simulink model "PCIe_UserLogic_00"  (Simulink 7.6)
settings: Solver=ode45  StartTime=0.0  StopTime=10.0  RelTol=1e-3
PreLoadFcn:
  | SP605_TS  = 1/200e6;
  | SP605_CLK = SP605_TS*1e9;
  | USER_TS  = 1/200e6;
  | USER_CLK = USER_TS*1e9;
  | 
  | PCIE_TS   = 1/125e6;
  | PCIE_CLK = PCIE_TS*1e9;
  | 
  | P_Size = 32;
  | 
  | WR_LAT = 10 + round(P_Size*5/12);
InitFcn:
  | SP605_TS  = 1/200e6;
  | SP605_CLK = SP605_TS*1e9;
  | USER_TS  = 1/200e6;
  | USER_CLK = USER_TS*1e9;
  | 
  | PCIE_TS   = 1/125e6;
  | PCIE_CLK = PCIE_TS*1e9;
  | 
  | P_Size = 32;
  | 
  | WR_LAT = 10 + round(P_Size*5/12);
libraries: xbsIndex_r4 x341
(part 3 of 3)

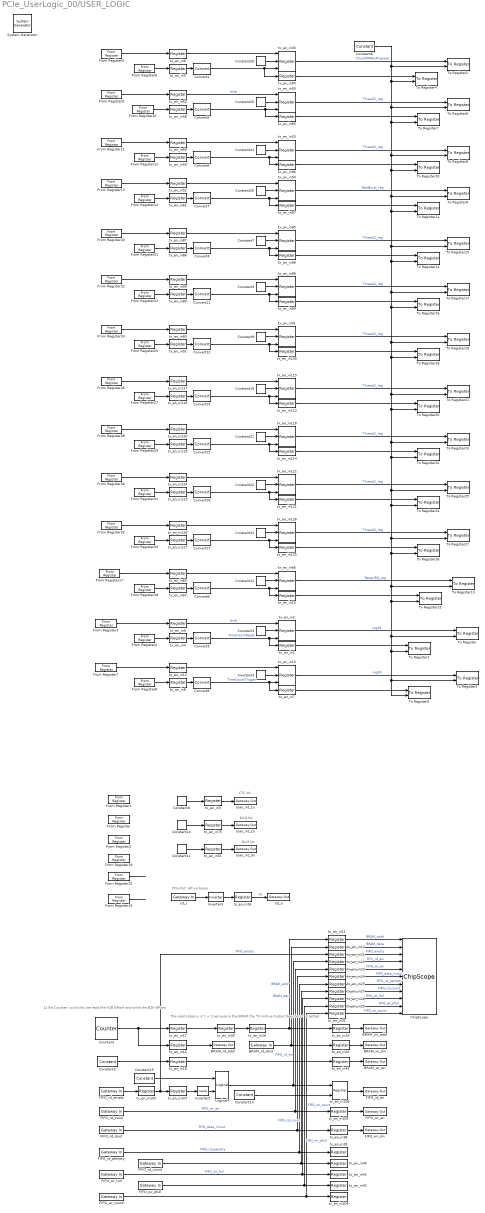
== system PCIe_UserLogic_00/USER_LOGIC ==
  note: The read Latency is 1 + 1 becouse
      | in the BRAM the "Primitive Output Registersr" is setted
  note: CTL bit
  note: DAQ bit
  note: DLM bit
  note: PCIe Rst: Attivo basso
  note: 12 Bit Counter:
      | cyclically we read the H2B BRam
      | and write the B2H BRam
  " System Generator" : xbsIndex_r4/ System Generator  Tag=genX  SystemSampleTime=-1  xilinxfamily=virtex6  part=xc6vlx240t  speed=-1  package=ff1156  synthesis_tool=XST  clock_wrapper=Clock Enables  directory=C:/Temp/Xilinx PCI Express/ML605_ISE13.3/MyUserLogic/UserLogic_00/top_level_1_PCIe_UserLogic_00_USER_LOGIC  proj_type=Project Navigator  Synth_file=XST Defaults  Impl_file=ISE Defaults  testbench=off  simulink_period=USER_TS  sysclk_period=USER_CLK  dcm_input_clock_period=5  incr_netlist=off  trim_vbits=Everywhere in SubSystem  dbl_ovrd=According to Block Masks  core_generation=According to Block Masks  run_coregen=off  deprecated_control=off  eval_field=0  block_type=sysgen
      settings: block_version=12.3
  BRAM_rd_addr : xbsIndex_r4/Gateway Out  hdl_port=on  timing_constraint=None  locs_specified=off  LOCs={}  block_type=gatewayout
      settings: infoedit="Gateway out block.  Converts Xilinx fixed point or floating-point type inputs into ouputs of type Simulink integer, double, or fixed point.<br><br>Hardware notes:  In hardware these blocks become top level output ports or are discarded, depending on how they are configured."  block_version=12.3
  BRAM_rd_dout : xbsIndex_r4/Gateway In  gui_display_data_type=Fixed-point  arith_type=Unsigned  n_bits=64  bin_pt=0  preci_type=Single  exp_width=8  frac_width=24  quantization="Round  (unbiased: +/- Inf)"  overflow=Saturate  period=USER_TS  dbl_ovrd=off  timing_constraint=None  locs_specified=off  LOCs={}  hdl_port=on  block_type=gatewayin
      settings: infoedit="Gateway in block.  Converts inputs of type Simulink integer, double and fixed point to  Xilinx fixed point type.<br><br>Hardware notes:  In hardware these blocks become top level input ports."  block_version=12.3
  BRAM_wr_addr : xbsIndex_r4/Gateway Out  hdl_port=on  timing_constraint=None  locs_specified=off  LOCs={}  block_type=gatewayout
      settings: infoedit="Gateway out block.  Converts Xilinx fixed point or floating-point type inputs into ouputs of type Simulink integer, double, or fixed point.<br><br>Hardware notes:  In hardware these blocks become top level output ports or are discarded, depending on how they are configured."  block_version=12.3
  BRAM_wr_din : xbsIndex_r4/Gateway Out  hdl_port=on  timing_constraint=None  locs_specified=off  LOCs={}  block_type=gatewayout
      settings: infoedit="Gateway out block.  Converts Xilinx fixed point or floating-point type inputs into ouputs of type Simulink integer, double, or fixed point.<br><br>Hardware notes:  In hardware these blocks become top level output ports or are discarded, depending on how they are configured."  block_version=12.3
  BRAM_wr_en : xbsIndex_r4/Gateway Out  hdl_port=on  timing_constraint=None  locs_specified=off  LOCs={}  block_type=gatewayout
      settings: infoedit="Gateway out block.  Converts Xilinx fixed point or floating-point type inputs into ouputs of type Simulink integer, double, or fixed point.<br><br>Hardware notes:  In hardware these blocks become top level output ports or are discarded, depending on how they are configured."  block_version=12.3
  ChipScope : xbsIndex_r4/ChipScope  num_trig_ports=11  current_port=0  show_trig_port=0  match_units=1  match_type=Basic  data_is_trigger=on  num_data_ports=1  data_depth=1024  SRL16s=on  add_bufg=on  match_type_t0=1  match_type_t1=1  match_type_t2=1  match_type_t3=1  match_type_t4=1  match_type_t5=1  match_type_t6=1  match_type_t7=1  match_type_t8=1  match_type_t9=1  match_type_t10=1  match_type_t11=1  match_type_t12=1  match_type_t13=1  match_type_t14=1  match_type_t15=1  match_units_t0=1  match_units_t1=1  match_units_t2=1  match_units_t3=1  match_units_t4=1  match_units_t5=1  match_units_t6=1  match_units_t7=1  match_units_t8=1  match_units_t9=1  match_units_t10=1  match_units_t11=1  match_units_t12=1  match_units_t13=1  match_units_t14=1  match_units_t15=1  dbl_ovrd=0  user_scan_chain=USER1  block_type=chipscope
      settings: infoedit="Enables run-time debugging and verification of signals by inserting ChipScope Pro ICON and ILA cores.<br><br>  Restrictions: <br>Only one ChipScope core can be instantiated in a System Generator design. A design or subsystem containing a ChipScope block must have at least one output port."
  Constant{1,3..4,7..12,19..26} (17 alike) : xbsIndex_r4/Constant  const=0  gui_display_data_type=Fixed-point  arith_type=Boolean  n_bits=32  bin_pt=0  preci_type=Single  exp_width=8  frac_width=24  explicit_period=on  period=USER_TS  equ=P=C  opselect=C  inp2=PCIN>>17  opr=+  inp1=P  carry=CIN  dbl_ovrd=off  block_type=constant
      settings: block_version=12.3
  Constant14 : xbsIndex_r4/Constant  const=1  gui_display_data_type=Fixed-point  arith_type=Boolean  n_bits=8  bin_pt=0  preci_type=Single  exp_width=8  frac_width=24  explicit_period=on  period=USER_TS  equ=P=C  opselect=C  inp2=PCIN>>17  opr=+  inp1=P  carry=CIN  dbl_ovrd=off  block_type=constant
      settings: block_version=12.3
  Constant15 : xbsIndex_r4/Constant  const=1  gui_display_data_type=Fixed-point  arith_type=Boolean  n_bits=8  bin_pt=0  preci_type=Single  exp_width=8  frac_width=24  explicit_period=on  period=USER_TS  equ=P=C  opselect=C  inp2=PCIN>>17  opr=+  inp1=P  carry=CIN  dbl_ovrd=off  block_type=constant
      settings: block_version=12.3
  Constant2 : xbsIndex_r4/Constant  const=255  gui_display_data_type=Fixed-point  arith_type=Unsigned  n_bits=8  bin_pt=0  preci_type=Single  exp_width=8  frac_width=24  explicit_period=on  period=USER_TS  equ=P=C  opselect=C  inp2=PCIN>>17  opr=+  inp1=P  carry=CIN  dbl_ovrd=off  block_type=constant
      settings: block_version=12.3
  Constant6 : xbsIndex_r4/Constant  const=1  gui_display_data_type=Fixed-point  arith_type=Boolean  n_bits=32  bin_pt=0  preci_type=Single  exp_width=8  frac_width=24  explicit_period=on  period=USER_TS  equ=P=C  opselect=C  inp2=PCIN>>17  opr=+  inp1=P  carry=CIN  dbl_ovrd=off  block_type=constant
      settings: block_version=12.3
  Convert{1,3..9,11..12,14..17} (14 alike) : xbsIndex_r4/Convert  gui_display_data_type=Fixed-point  arith_type=Boolean  n_bits=16  bin_pt=14  float_type=Single  exp_bits=8  fraction_bits=24  quantization=Truncate  overflow=Wrap  en=off  latency=0  dbl_ovrd=off  pipeline=off  block_type=convert
      settings: block_version=12.3
  Counter4 : xbsIndex_r4/Counter  cnt_type=Free Running  cnt_to=Inf  operation=Up  start_count=0  cnt_by_val=1  arith_type=Unsigned  n_bits=12  bin_pt=0  load_pin=off  rst=off  en=off  explicit_period=on  period=USER_TS  dbl_ovrd=off  use_behavioral_HDL=off  implementation=Fabric  block_type=counter
      settings: block_version=12.3
  FIFO_rd_count : xbsIndex_r4/Gateway In  gui_display_data_type=Fixed-point  arith_type=Unsigned  n_bits=15  bin_pt=0  preci_type=Single  exp_width=8  frac_width=24  quantization="Round  (unbiased: +/- Inf)"  overflow=Saturate  period=USER_TS  dbl_ovrd=off  timing_constraint=None  locs_specified=off  LOCs={}  hdl_port=on  block_type=gatewayin
      settings: infoedit="Gateway in block.  Converts inputs of type Simulink integer, double and fixed point to  Xilinx fixed point type.<br><br>Hardware notes:  In hardware these blocks become top level input ports."  block_version=12.3
  FIFO_rd_dout : xbsIndex_r4/Gateway In  gui_display_data_type=Fixed-point  arith_type=Unsigned  n_bits=72  bin_pt=0  preci_type=Single  exp_width=8  frac_width=24  quantization="Round  (unbiased: +/- Inf)"  overflow=Saturate  period=USER_TS  dbl_ovrd=off  timing_constraint=None  locs_specified=off  LOCs={}  hdl_port=on  block_type=gatewayin
      settings: infoedit="Gateway in block.  Converts inputs of type Simulink integer, double and fixed point to  Xilinx fixed point type.<br><br>Hardware notes:  In hardware these blocks become top level input ports."  block_version=12.3
  FIFO_rd_empty : xbsIndex_r4/Gateway In  gui_display_data_type=Fixed-point  arith_type=Boolean  n_bits=12  bin_pt=0  preci_type=Single  exp_width=8  frac_width=24  quantization="Round  (unbiased: +/- Inf)"  overflow=Saturate  period=USER_TS  dbl_ovrd=off  timing_constraint=None  locs_specified=off  LOCs={}  hdl_port=on  block_type=gatewayin
      settings: infoedit="Gateway in block.  Converts inputs of type Simulink integer, double and fixed point to  Xilinx fixed point type.<br><br>Hardware notes:  In hardware these blocks become top level input ports."  block_version=12.3
  FIFO_rd_en : xbsIndex_r4/Gateway Out  hdl_port=on  timing_constraint=None  locs_specified=off  LOCs={}  block_type=gatewayout
      settings: infoedit="Gateway out block.  Converts Xilinx fixed point or floating-point type inputs into ouputs of type Simulink integer, double, or fixed point.<br><br>Hardware notes:  In hardware these blocks become top level output ports or are discarded, depending on how they are configured."  block_version=12.3
  FIFO_rd_pempty : xbsIndex_r4/Gateway In  gui_display_data_type=Fixed-point  arith_type=Boolean  n_bits=64  bin_pt=0  preci_type=Single  exp_width=8  frac_width=24  quantization="Round  (unbiased: +/- Inf)"  overflow=Saturate  period=USER_TS  dbl_ovrd=off  timing_constraint=None  locs_specified=off  LOCs={}  hdl_port=on  block_type=gatewayin
      settings: infoedit="Gateway in block.  Converts inputs of type Simulink integer, double and fixed point to  Xilinx fixed point type.<br><br>Hardware notes:  In hardware these blocks become top level input ports."  block_version=12.3
  FIFO_rd_valid : xbsIndex_r4/Gateway In  gui_display_data_type=Fixed-point  arith_type=Boolean  n_bits=14  bin_pt=0  preci_type=Single  exp_width=8  frac_width=24  quantization="Round  (unbiased: +/- Inf)"  overflow=Saturate  period=USER_TS  dbl_ovrd=off  timing_constraint=None  locs_specified=off  LOCs={}  hdl_port=on  block_type=gatewayin
      settings: infoedit="Gateway in block.  Converts inputs of type Simulink integer, double and fixed point to  Xilinx fixed point type.<br><br>Hardware notes:  In hardware these blocks become top level input ports."  block_version=12.3
  FIFO_wr_count : xbsIndex_r4/Gateway In  gui_display_data_type=Fixed-point  arith_type=Unsigned  n_bits=15  bin_pt=0  preci_type=Single  exp_width=8  frac_width=24  quantization="Round  (unbiased: +/- Inf)"  overflow=Saturate  period=USER_TS  dbl_ovrd=off  timing_constraint=None  locs_specified=off  LOCs={}  hdl_port=on  block_type=gatewayin
      settings: infoedit="Gateway in block.  Converts inputs of type Simulink integer, double and fixed point to  Xilinx fixed point type.<br><br>Hardware notes:  In hardware these blocks become top level input ports."  block_version=12.3
  FIFO_wr_din : xbsIndex_r4/Gateway Out  hdl_port=on  timing_constraint=None  locs_specified=off  LOCs={}  block_type=gatewayout
      settings: infoedit="Gateway out block.  Converts Xilinx fixed point or floating-point type inputs into ouputs of type Simulink integer, double, or fixed point.<br><br>Hardware notes:  In hardware these blocks become top level output ports or are discarded, depending on how they are configured."  block_version=12.3
  FIFO_wr_en : xbsIndex_r4/Gateway Out  hdl_port=on  timing_constraint=None  locs_specified=off  LOCs={}  block_type=gatewayout
      settings: infoedit="Gateway out block.  Converts Xilinx fixed point or floating-point type inputs into ouputs of type Simulink integer, double, or fixed point.<br><br>Hardware notes:  In hardware these blocks become top level output ports or are discarded, depending on how they are configured."  block_version=12.3
  FIFO_wr_full : xbsIndex_r4/Gateway In  gui_display_data_type=Fixed-point  arith_type=Boolean  n_bits=8  bin_pt=0  preci_type=Single  exp_width=8  frac_width=24  quantization="Round  (unbiased: +/- Inf)"  overflow=Saturate  period=USER_TS  dbl_ovrd=off  timing_constraint=None  locs_specified=off  LOCs={}  hdl_port=on  block_type=gatewayin
      settings: infoedit="Gateway in block.  Converts inputs of type Simulink integer, double and fixed point to  Xilinx fixed point type.<br><br>Hardware notes:  In hardware these blocks become top level input ports."  block_version=12.3
  FIFO_wr_pfull : xbsIndex_r4/Gateway In  gui_display_data_type=Fixed-point  arith_type=Boolean  n_bits=64  bin_pt=0  preci_type=Single  exp_width=8  frac_width=24  quantization="Round  (unbiased: +/- Inf)"  overflow=Saturate  period=USER_TS  dbl_ovrd=off  timing_constraint=None  locs_specified=off  LOCs={}  hdl_port=on  block_type=gatewayin
      settings: infoedit="Gateway in block.  Converts inputs of type Simulink integer, double and fixed point to  Xilinx fixed point type.<br><br>Hardware notes:  In hardware these blocks become top level input ports."  block_version=12.3
  From Register : xbsIndex_r4/From Register  shared_memory_name='debug1i'  init=0  period=USER_TS  ownership=Owned and initialized elsewhere  gui_display_data_type=Fixed-point  arith_type=Unsigned  n_bits=32  bin_pt=0  preci_type=Single  dbl_ovrd=off  block_type=fromreg
      settings: AttributesFormatString=<< %<shared_memory_name> >>  infoedit="Register block that reads data to a shared memory register.  Delay of one sample period."  block_version=12.3
  From Register1 : xbsIndex_r4/From Register  shared_memory_name='debug2i'  init=0  period=USER_TS  ownership=Owned and initialized elsewhere  gui_display_data_type=Fixed-point  arith_type=Unsigned  n_bits=32  bin_pt=0  preci_type=Single  dbl_ovrd=off  block_type=fromreg
      settings: AttributesFormatString=<< %<shared_memory_name> >>  infoedit="Register block that reads data to a shared memory register.  Delay of one sample period."  block_version=12.3
  From Register10 : xbsIndex_r4/From Register  shared_memory_name='register04tv'  init=0  period=USER_TS  ownership=Owned and initialized elsewhere  gui_display_data_type=Fixed-point  arith_type=Unsigned  n_bits=1  bin_pt=0  preci_type=Single  dbl_ovrd=off  block_type=fromreg
      settings: AttributesFormatString=<< %<shared_memory_name> >>  infoedit="Register block that reads data to a shared memory register.  Delay of one sample period."  block_version=12.3
  From Register11 : xbsIndex_r4/From Register  shared_memory_name='register05td'  init=0  period=USER_TS  ownership=Owned and initialized elsewhere  gui_display_data_type=Fixed-point  arith_type=Unsigned  n_bits=32  bin_pt=0  preci_type=Single  dbl_ovrd=off  block_type=fromreg
      settings: AttributesFormatString=<< %<shared_memory_name> >>  infoedit="Register block that reads data to a shared memory register.  Delay of one sample period."  block_version=12.3
  From Register12 : xbsIndex_r4/From Register  shared_memory_name='register05tv'  init=0  period=USER_TS  ownership=Owned and initialized elsewhere  gui_display_data_type=Fixed-point  arith_type=Unsigned  n_bits=1  bin_pt=0  preci_type=Single  dbl_ovrd=off  block_type=fromreg
      settings: AttributesFormatString=<< %<shared_memory_name> >>  infoedit="Register block that reads data to a shared memory register.  Delay of one sample period."  block_version=12.3
  From Register13 : xbsIndex_r4/From Register  shared_memory_name='register06td'  init=0  period=USER_TS  ownership=Owned and initialized elsewhere  gui_display_data_type=Fixed-point  arith_type=Unsigned  n_bits=32  bin_pt=0  preci_type=Single  dbl_ovrd=off  block_type=fromreg
      settings: AttributesFormatString=<< %<shared_memory_name> >>  infoedit="Register block that reads data to a shared memory register.  Delay of one sample period."  block_version=12.3
  From Register14 : xbsIndex_r4/From Register  shared_memory_name='register06tv'  init=0  period=USER_TS  ownership=Owned and initialized elsewhere  gui_display_data_type=Fixed-point  arith_type=Unsigned  n_bits=1  bin_pt=0  preci_type=Single  dbl_ovrd=off  block_type=fromreg
      settings: AttributesFormatString=<< %<shared_memory_name> >>  infoedit="Register block that reads data to a shared memory register.  Delay of one sample period."  block_version=12.3
  From Register15 : xbsIndex_r4/From Register  shared_memory_name='DMA_Host2Board_Done'  init=0  period=USER_TS  ownership=Owned and initialized elsewhere  gui_display_data_type=Fixed-point  arith_type=Unsigned  n_bits=1  bin_pt=0  preci_type=Single  dbl_ovrd=off  block_type=fromreg
      settings: AttributesFormatString=<< %<shared_memory_name> >>  infoedit="Register block that reads data to a shared memory register.  Delay of one sample period."  block_version=12.3
  From Register16 : xbsIndex_r4/From Register  shared_memory_name='DMA_Host2Board_Busy'  init=0  period=USER_TS  ownership=Owned and initialized elsewhere  gui_display_data_type=Fixed-point  arith_type=Unsigned  n_bits=1  bin_pt=0  preci_type=Single  dbl_ovrd=off  block_type=fromreg
      settings: AttributesFormatString=<< %<shared_memory_name> >>  infoedit="Register block that reads data to a shared memory register.  Delay of one sample period."  block_version=12.3
  From Register17 : xbsIndex_r4/From Register  shared_memory_name='register07td'  init=0  period=USER_TS  ownership=Owned and initialized elsewhere  gui_display_data_type=Fixed-point  arith_type=Unsigned  n_bits=32  bin_pt=0  preci_type=Single  dbl_ovrd=off  block_type=fromreg
      settings: AttributesFormatString=<< %<shared_memory_name> >>  infoedit="Register block that reads data to a shared memory register.  Delay of one sample period."  block_version=12.3
  From Register18 : xbsIndex_r4/From Register  shared_memory_name='register07tv'  init=0  period=USER_TS  ownership=Owned and initialized elsewhere  gui_display_data_type=Fixed-point  arith_type=Unsigned  n_bits=1  bin_pt=0  preci_type=Single  dbl_ovrd=off  block_type=fromreg
      settings: AttributesFormatString=<< %<shared_memory_name> >>  infoedit="Register block that reads data to a shared memory register.  Delay of one sample period."  block_version=12.3
  From Register19 : xbsIndex_r4/From Register  shared_memory_name='debug4i'  init=0  period=USER_TS  ownership=Owned and initialized elsewhere  gui_display_data_type=Fixed-point  arith_type=Unsigned  n_bits=32  bin_pt=0  preci_type=Single  dbl_ovrd=off  block_type=fromreg
      settings: AttributesFormatString=<< %<shared_memory_name> >>  infoedit="Register block that reads data to a shared memory register.  Delay of one sample period."  block_version=12.3
  From Register2 : xbsIndex_r4/From Register  shared_memory_name='debug3i'  init=0  period=USER_TS  ownership=Owned and initialized elsewhere  gui_display_data_type=Fixed-point  arith_type=Unsigned  n_bits=32  bin_pt=0  preci_type=Single  dbl_ovrd=off  block_type=fromreg
      settings: AttributesFormatString=<< %<shared_memory_name> >>  infoedit="Register block that reads data to a shared memory register.  Delay of one sample period."  block_version=12.3
  From Register20 : xbsIndex_r4/From Register  shared_memory_name='register08td'  init=0  period=USER_TS  ownership=Owned and initialized elsewhere  gui_display_data_type=Fixed-point  arith_type=Unsigned  n_bits=32  bin_pt=0  preci_type=Single  dbl_ovrd=off  block_type=fromreg
      settings: AttributesFormatString=<< %<shared_memory_name> >>  infoedit="Register block that reads data to a shared memory register.  Delay of one sample period."  block_version=12.3
  From Register21 : xbsIndex_r4/From Register  shared_memory_name='register08tv'  init=0  period=USER_TS  ownership=Owned and initialized elsewhere  gui_display_data_type=Fixed-point  arith_type=Unsigned  n_bits=1  bin_pt=0  preci_type=Single  dbl_ovrd=off  block_type=fromreg
      settings: AttributesFormatString=<< %<shared_memory_name> >>  infoedit="Register block that reads data to a shared memory register.  Delay of one sample period."  block_version=12.3
  From Register22 : xbsIndex_r4/From Register  shared_memory_name='register09td'  init=0  period=USER_TS  ownership=Owned and initialized elsewhere  gui_display_data_type=Fixed-point  arith_type=Unsigned  n_bits=32  bin_pt=0  preci_type=Single  dbl_ovrd=off  block_type=fromreg
      settings: AttributesFormatString=<< %<shared_memory_name> >>  infoedit="Register block that reads data to a shared memory register.  Delay of one sample period."  block_version=12.3
  From Register23 : xbsIndex_r4/From Register  shared_memory_name='register09tv'  init=0  period=USER_TS  ownership=Owned and initialized elsewhere  gui_display_data_type=Fixed-point  arith_type=Unsigned  n_bits=1  bin_pt=0  preci_type=Single  dbl_ovrd=off  block_type=fromreg
      settings: AttributesFormatString=<< %<shared_memory_name> >>  infoedit="Register block that reads data to a shared memory register.  Delay of one sample period."  block_version=12.3
  From Register24 : xbsIndex_r4/From Register  shared_memory_name='register10td'  init=0  period=USER_TS  ownership=Owned and initialized elsewhere  gui_display_data_type=Fixed-point  arith_type=Unsigned  n_bits=32  bin_pt=0  preci_type=Single  dbl_ovrd=off  block_type=fromreg
      settings: AttributesFormatString=<< %<shared_memory_name> >>  infoedit="Register block that reads data to a shared memory register.  Delay of one sample period."  block_version=12.3
  From Register25 : xbsIndex_r4/From Register  shared_memory_name='register10tv'  init=0  period=USER_TS  ownership=Owned and initialized elsewhere  gui_display_data_type=Fixed-point  arith_type=Unsigned  n_bits=1  bin_pt=0  preci_type=Single  dbl_ovrd=off  block_type=fromreg
      settings: AttributesFormatString=<< %<shared_memory_name> >>  infoedit="Register block that reads data to a shared memory register.  Delay of one sample period."  block_version=12.3
  From Register26 : xbsIndex_r4/From Register  shared_memory_name='register11td'  init=0  period=USER_TS  ownership=Owned and initialized elsewhere  gui_display_data_type=Fixed-point  arith_type=Unsigned  n_bits=32  bin_pt=0  preci_type=Single  dbl_ovrd=off  block_type=fromreg
      settings: AttributesFormatString=<< %<shared_memory_name> >>  infoedit="Register block that reads data to a shared memory register.  Delay of one sample period."  block_version=12.3
  From Register27 : xbsIndex_r4/From Register  shared_memory_name='register11tv'  init=0  period=USER_TS  ownership=Owned and initialized elsewhere  gui_display_data_type=Fixed-point  arith_type=Unsigned  n_bits=1  bin_pt=0  preci_type=Single  dbl_ovrd=off  block_type=fromreg
      settings: AttributesFormatString=<< %<shared_memory_name> >>  infoedit="Register block that reads data to a shared memory register.  Delay of one sample period."  block_version=12.3
  From Register28 : xbsIndex_r4/From Register  shared_memory_name='register12td'  init=0  period=USER_TS  ownership=Owned and initialized elsewhere  gui_display_data_type=Fixed-point  arith_type=Unsigned  n_bits=32  bin_pt=0  preci_type=Single  dbl_ovrd=off  block_type=fromreg
      settings: AttributesFormatString=<< %<shared_memory_name> >>  infoedit="Register block that reads data to a shared memory register.  Delay of one sample period."  block_version=12.3
  From Register29 : xbsIndex_r4/From Register  shared_memory_name='register12tv'  init=0  period=USER_TS  ownership=Owned and initialized elsewhere  gui_display_data_type=Fixed-point  arith_type=Unsigned  n_bits=1  bin_pt=0  preci_type=Single  dbl_ovrd=off  block_type=fromreg
      settings: AttributesFormatString=<< %<shared_memory_name> >>  infoedit="Register block that reads data to a shared memory register.  Delay of one sample period."  block_version=12.3
  From Register3 : xbsIndex_r4/From Register  shared_memory_name='register01td'  init=0  period=USER_TS  ownership=Owned and initialized elsewhere  gui_display_data_type=Fixed-point  arith_type=Unsigned  n_bits=32  bin_pt=0  preci_type=Single  dbl_ovrd=off  block_type=fromreg
      settings: AttributesFormatString=<< %<shared_memory_name> >>  infoedit="Register block that reads data to a shared memory register.  Delay of one sample period."  block_version=12.3
  From Register30 : xbsIndex_r4/From Register  shared_memory_name='register13td'  init=0  period=USER_TS  ownership=Owned and initialized elsewhere  gui_display_data_type=Fixed-point  arith_type=Unsigned  n_bits=32  bin_pt=0  preci_type=Single  dbl_ovrd=off  block_type=fromreg
      settings: AttributesFormatString=<< %<shared_memory_name> >>  infoedit="Register block that reads data to a shared memory register.  Delay of one sample period."  block_version=12.3
  From Register31 : xbsIndex_r4/From Register  shared_memory_name='register13tv'  init=0  period=USER_TS  ownership=Owned and initialized elsewhere  gui_display_data_type=Fixed-point  arith_type=Unsigned  n_bits=1  bin_pt=0  preci_type=Single  dbl_ovrd=off  block_type=fromreg
      settings: AttributesFormatString=<< %<shared_memory_name> >>  infoedit="Register block that reads data to a shared memory register.  Delay of one sample period."  block_version=12.3
  From Register32 : xbsIndex_r4/From Register  shared_memory_name='register14td'  init=0  period=USER_TS  ownership=Owned and initialized elsewhere  gui_display_data_type=Fixed-point  arith_type=Unsigned  n_bits=32  bin_pt=0  preci_type=Single  dbl_ovrd=off  block_type=fromreg
      settings: AttributesFormatString=<< %<shared_memory_name> >>  infoedit="Register block that reads data to a shared memory register.  Delay of one sample period."  block_version=12.3
  From Register33 : xbsIndex_r4/From Register  shared_memory_name='register14tv'  init=0  period=USER_TS  ownership=Owned and initialized elsewhere  gui_display_data_type=Fixed-point  arith_type=Unsigned  n_bits=1  bin_pt=0  preci_type=Single  dbl_ovrd=off  block_type=fromreg
      settings: AttributesFormatString=<< %<shared_memory_name> >>  infoedit="Register block that reads data to a shared memory register.  Delay of one sample period."  block_version=12.3
  From Register4 : xbsIndex_r4/From Register  shared_memory_name='register01tv'  init=0  period=USER_TS  ownership=Owned and initialized elsewhere  gui_display_data_type=Fixed-point  arith_type=Unsigned  n_bits=1  bin_pt=0  preci_type=Single  dbl_ovrd=off  block_type=fromreg
      settings: AttributesFormatString=<< %<shared_memory_name> >>  infoedit="Register block that reads data to a shared memory register.  Delay of one sample period."  block_version=12.3
  From Register5 : xbsIndex_r4/From Register  shared_memory_name='register02td'  init=0  period=USER_TS  ownership=Owned and initialized elsewhere  gui_display_data_type=Fixed-point  arith_type=Unsigned  n_bits=32  bin_pt=0  preci_type=Single  dbl_ovrd=off  block_type=fromreg
      settings: AttributesFormatString=<< %<shared_memory_name> >>  infoedit="Register block that reads data to a shared memory register.  Delay of one sample period."  block_version=12.3
  From Register6 : xbsIndex_r4/From Register  shared_memory_name='register02tv'  init=0  period=USER_TS  ownership=Owned and initialized elsewhere  gui_display_data_type=Fixed-point  arith_type=Unsigned  n_bits=1  bin_pt=0  preci_type=Single  dbl_ovrd=off  block_type=fromreg
      settings: AttributesFormatString=<< %<shared_memory_name> >>  infoedit="Register block that reads data to a shared memory register.  Delay of one sample period."  block_version=12.3
  From Register7 : xbsIndex_r4/From Register  shared_memory_name='register03td'  init=0  period=USER_TS  ownership=Owned and initialized elsewhere  gui_display_data_type=Fixed-point  arith_type=Unsigned  n_bits=32  bin_pt=0  preci_type=Single  dbl_ovrd=off  block_type=fromreg
      settings: AttributesFormatString=<< %<shared_memory_name> >>  infoedit="Register block that reads data to a shared memory register.  Delay of one sample period."  block_version=12.3
  From Register8 : xbsIndex_r4/From Register  shared_memory_name='register03tv'  init=0  period=USER_TS  ownership=Owned and initialized elsewhere  gui_display_data_type=Fixed-point  arith_type=Unsigned  n_bits=1  bin_pt=0  preci_type=Single  dbl_ovrd=off  block_type=fromreg
      settings: AttributesFormatString=<< %<shared_memory_name> >>  infoedit="Register block that reads data to a shared memory register.  Delay of one sample period."  block_version=12.3
  From Register9 : xbsIndex_r4/From Register  shared_memory_name='register04td'  init=0  period=USER_TS  ownership=Owned and initialized elsewhere  gui_display_data_type=Fixed-point  arith_type=Unsigned  n_bits=32  bin_pt=0  preci_type=Single  dbl_ovrd=off  block_type=fromreg
      settings: AttributesFormatString=<< %<shared_memory_name> >>  infoedit="Register block that reads data to a shared memory register.  Delay of one sample period."  block_version=12.3
  Inverter3 : xbsIndex_r4/Inverter  en=off  latency=0  dbl_ovrd=off  block_type=inv
      settings: block_version=12.3
  Inverter5 : xbsIndex_r4/Inverter  en=off  latency=0  dbl_ovrd=off  block_type=inv
      settings: block_version=12.3
  Logical4 : xbsIndex_r4/Logical  logical_function=AND  inputs=2  en=off  latency=0  precision=Full  arith_type=Unsigned  n_bits=16  bin_pt=0  align_bp=on  dbl_ovrd=off  block_type=logical
      settings: block_version=12.3
  To Register : xbsIndex_r4/To Register  shared_memory_name='register01rd'  init=0  ownership=Locally owned and initialized  explicit_data_type=off  gui_display_data_type=Fixed-point  arith_type="Signed  (2's comp)"  n_bits=16  bin_pt=14  preci_type=Single  dbl_ovrd=off  block_type=toreg
      settings: AttributesFormatString=<< %<shared_memory_name> >>  infoedit="Register block that writes data to a shared memory register.  Delay of one sample period."  block_version=12.3
  To Register1 : xbsIndex_r4/To Register  shared_memory_name='register01rv'  init=0  ownership=Locally owned and initialized  explicit_data_type=off  gui_display_data_type=Fixed-point  arith_type="Signed  (2's comp)"  n_bits=16  bin_pt=14  preci_type=Single  dbl_ovrd=off  block_type=toreg
      settings: AttributesFormatString=<< %<shared_memory_name> >>  infoedit="Register block that writes data to a shared memory register.  Delay of one sample period."  block_version=12.3
  To Register10 : xbsIndex_r4/To Register  shared_memory_name='register05rv'  init=0  ownership=Locally owned and initialized  explicit_data_type=off  gui_display_data_type=Fixed-point  arith_type="Signed  (2's comp)"  n_bits=16  bin_pt=14  preci_type=Single  dbl_ovrd=off  block_type=toreg
      settings: AttributesFormatString=<< %<shared_memory_name> >>  infoedit="Register block that writes data to a shared memory register.  Delay of one sample period."  block_version=12.3
  To Register11 : xbsIndex_r4/To Register  shared_memory_name='register06rv'  init=0  ownership=Locally owned and initialized  explicit_data_type=off  gui_display_data_type=Fixed-point  arith_type="Signed  (2's comp)"  n_bits=16  bin_pt=14  preci_type=Single  dbl_ovrd=off  block_type=toreg
      settings: AttributesFormatString=<< %<shared_memory_name> >>  infoedit="Register block that writes data to a shared memory register.  Delay of one sample period."  block_version=12.3
  To Register12 : xbsIndex_r4/To Register  shared_memory_name='register07rv'  init=0  ownership=Locally owned and initialized  explicit_data_type=off  gui_display_data_type=Fixed-point  arith_type="Signed  (2's comp)"  n_bits=16  bin_pt=14  preci_type=Single  dbl_ovrd=off  block_type=toreg
      settings: AttributesFormatString=<< %<shared_memory_name> >>  infoedit="Register block that writes data to a shared memory register.  Delay of one sample period."  block_version=12.3
  To Register13 : xbsIndex_r4/To Register  shared_memory_name='register07rd'  init=0  ownership=Locally owned and initialized  explicit_data_type=off  gui_display_data_type=Fixed-point  arith_type="Signed  (2's comp)"  n_bits=16  bin_pt=14  preci_type=Single  dbl_ovrd=off  block_type=toreg
      settings: AttributesFormatString=<< %<shared_memory_name> >>  infoedit="Register block that writes data to a shared memory register.  Delay of one sample period."  block_version=12.3
  To Register14 : xbsIndex_r4/To Register  shared_memory_name='register08rv'  init=0  ownership=Locally owned and initialized  explicit_data_type=off  gui_display_data_type=Fixed-point  arith_type="Signed  (2's comp)"  n_bits=16  bin_pt=14  preci_type=Single  dbl_ovrd=off  block_type=toreg
      settings: AttributesFormatString=<< %<shared_memory_name> >>  infoedit="Register block that writes data to a shared memory register.  Delay of one sample period."  block_version=12.3
  To Register15 : xbsIndex_r4/To Register  shared_memory_name='register08rd'  init=0  ownership=Locally owned and initialized  explicit_data_type=off  gui_display_data_type=Fixed-point  arith_type="Signed  (2's comp)"  n_bits=16  bin_pt=14  preci_type=Single  dbl_ovrd=off  block_type=toreg
      settings: AttributesFormatString=<< %<shared_memory_name> >>  infoedit="Register block that writes data to a shared memory register.  Delay of one sample period."  block_version=12.3
  To Register16 : xbsIndex_r4/To Register  shared_memory_name='register09rv'  init=0  ownership=Locally owned and initialized  explicit_data_type=off  gui_display_data_type=Fixed-point  arith_type="Signed  (2's comp)"  n_bits=16  bin_pt=14  preci_type=Single  dbl_ovrd=off  block_type=toreg
      settings: AttributesFormatString=<< %<shared_memory_name> >>  infoedit="Register block that writes data to a shared memory register.  Delay of one sample period."  block_version=12.3
  To Register17 : xbsIndex_r4/To Register  shared_memory_name='register09rd'  init=0  ownership=Locally owned and initialized  explicit_data_type=off  gui_display_data_type=Fixed-point  arith_type="Signed  (2's comp)"  n_bits=16  bin_pt=14  preci_type=Single  dbl_ovrd=off  block_type=toreg
      settings: AttributesFormatString=<< %<shared_memory_name> >>  infoedit="Register block that writes data to a shared memory register.  Delay of one sample period."  block_version=12.3
  To Register18 : xbsIndex_r4/To Register  shared_memory_name='register10rv'  init=0  ownership=Locally owned and initialized  explicit_data_type=off  gui_display_data_type=Fixed-point  arith_type="Signed  (2's comp)"  n_bits=16  bin_pt=14  preci_type=Single  dbl_ovrd=off  block_type=toreg
      settings: AttributesFormatString=<< %<shared_memory_name> >>  infoedit="Register block that writes data to a shared memory register.  Delay of one sample period."  block_version=12.3
  To Register19 : xbsIndex_r4/To Register  shared_memory_name='register10rd'  init=0  ownership=Locally owned and initialized  explicit_data_type=off  gui_display_data_type=Fixed-point  arith_type="Signed  (2's comp)"  n_bits=16  bin_pt=14  preci_type=Single  dbl_ovrd=off  block_type=toreg
      settings: AttributesFormatString=<< %<shared_memory_name> >>  infoedit="Register block that writes data to a shared memory register.  Delay of one sample period."  block_version=12.3
  To Register2 : xbsIndex_r4/To Register  shared_memory_name='register02rd'  init=0  ownership=Locally owned and initialized  explicit_data_type=off  gui_display_data_type=Fixed-point  arith_type="Signed  (2's comp)"  n_bits=16  bin_pt=14  preci_type=Single  dbl_ovrd=off  block_type=toreg
      settings: AttributesFormatString=<< %<shared_memory_name> >>  infoedit="Register block that writes data to a shared memory register.  Delay of one sample period."  block_version=12.3
  To Register20 : xbsIndex_r4/To Register  shared_memory_name='register11rv'  init=0  ownership=Locally owned and initialized  explicit_data_type=off  gui_display_data_type=Fixed-point  arith_type="Signed  (2's comp)"  n_bits=16  bin_pt=14  preci_type=Single  dbl_ovrd=off  block_type=toreg
      settings: AttributesFormatString=<< %<shared_memory_name> >>  infoedit="Register block that writes data to a shared memory register.  Delay of one sample period."  block_version=12.3
  To Register21 : xbsIndex_r4/To Register  shared_memory_name='register11rd'  init=0  ownership=Locally owned and initialized  explicit_data_type=off  gui_display_data_type=Fixed-point  arith_type="Signed  (2's comp)"  n_bits=16  bin_pt=14  preci_type=Single  dbl_ovrd=off  block_type=toreg
      settings: AttributesFormatString=<< %<shared_memory_name> >>  infoedit="Register block that writes data to a shared memory register.  Delay of one sample period."  block_version=12.3
  To Register22 : xbsIndex_r4/To Register  shared_memory_name='register12rv'  init=0  ownership=Locally owned and initialized  explicit_data_type=off  gui_display_data_type=Fixed-point  arith_type="Signed  (2's comp)"  n_bits=16  bin_pt=14  preci_type=Single  dbl_ovrd=off  block_type=toreg
      settings: AttributesFormatString=<< %<shared_memory_name> >>  infoedit="Register block that writes data to a shared memory register.  Delay of one sample period."  block_version=12.3
  To Register23 : xbsIndex_r4/To Register  shared_memory_name='register12rd'  init=0  ownership=Locally owned and initialized  explicit_data_type=off  gui_display_data_type=Fixed-point  arith_type="Signed  (2's comp)"  n_bits=16  bin_pt=14  preci_type=Single  dbl_ovrd=off  block_type=toreg
      settings: AttributesFormatString=<< %<shared_memory_name> >>  infoedit="Register block that writes data to a shared memory register.  Delay of one sample period."  block_version=12.3
  To Register24 : xbsIndex_r4/To Register  shared_memory_name='register13rv'  init=0  ownership=Locally owned and initialized  explicit_data_type=off  gui_display_data_type=Fixed-point  arith_type="Signed  (2's comp)"  n_bits=16  bin_pt=14  preci_type=Single  dbl_ovrd=off  block_type=toreg
      settings: AttributesFormatString=<< %<shared_memory_name> >>  infoedit="Register block that writes data to a shared memory register.  Delay of one sample period."  block_version=12.3
  To Register25 : xbsIndex_r4/To Register  shared_memory_name='register13rd'  init=0  ownership=Locally owned and initialized  explicit_data_type=off  gui_display_data_type=Fixed-point  arith_type="Signed  (2's comp)"  n_bits=16  bin_pt=14  preci_type=Single  dbl_ovrd=off  block_type=toreg
      settings: AttributesFormatString=<< %<shared_memory_name> >>  infoedit="Register block that writes data to a shared memory register.  Delay of one sample period."  block_version=12.3
  To Register26 : xbsIndex_r4/To Register  shared_memory_name='register14rv'  init=0  ownership=Locally owned and initialized  explicit_data_type=off  gui_display_data_type=Fixed-point  arith_type="Signed  (2's comp)"  n_bits=16  bin_pt=14  preci_type=Single  dbl_ovrd=off  block_type=toreg
      settings: AttributesFormatString=<< %<shared_memory_name> >>  infoedit="Register block that writes data to a shared memory register.  Delay of one sample period."  block_version=12.3
  To Register27 : xbsIndex_r4/To Register  shared_memory_name='register14rd'  init=0  ownership=Locally owned and initialized  explicit_data_type=off  gui_display_data_type=Fixed-point  arith_type="Signed  (2's comp)"  n_bits=16  bin_pt=14  preci_type=Single  dbl_ovrd=off  block_type=toreg
      settings: AttributesFormatString=<< %<shared_memory_name> >>  infoedit="Register block that writes data to a shared memory register.  Delay of one sample period."  block_version=12.3
  To Register3 : xbsIndex_r4/To Register  shared_memory_name='register03rd'  init=0  ownership=Locally owned and initialized  explicit_data_type=off  gui_display_data_type=Fixed-point  arith_type="Signed  (2's comp)"  n_bits=16  bin_pt=14  preci_type=Single  dbl_ovrd=off  block_type=toreg
      settings: AttributesFormatString=<< %<shared_memory_name> >>  infoedit="Register block that writes data to a shared memory register.  Delay of one sample period."  block_version=12.3
  To Register4 : xbsIndex_r4/To Register  shared_memory_name='register02rv'  init=0  ownership=Locally owned and initialized  explicit_data_type=off  gui_display_data_type=Fixed-point  arith_type="Signed  (2's comp)"  n_bits=16  bin_pt=14  preci_type=Single  dbl_ovrd=off  block_type=toreg
      settings: AttributesFormatString=<< %<shared_memory_name> >>  infoedit="Register block that writes data to a shared memory register.  Delay of one sample period."  block_version=12.3
  To Register5 : xbsIndex_r4/To Register  shared_memory_name='register03rv'  init=0  ownership=Locally owned and initialized  explicit_data_type=off  gui_display_data_type=Fixed-point  arith_type="Signed  (2's comp)"  n_bits=16  bin_pt=14  preci_type=Single  dbl_ovrd=off  block_type=toreg
      settings: AttributesFormatString=<< %<shared_memory_name> >>  infoedit="Register block that writes data to a shared memory register.  Delay of one sample period."  block_version=12.3
  To Register6 : xbsIndex_r4/To Register  shared_memory_name='register04rd'  init=0  ownership=Locally owned and initialized  explicit_data_type=off  gui_display_data_type=Fixed-point  arith_type="Signed  (2's comp)"  n_bits=16  bin_pt=14  preci_type=Single  dbl_ovrd=off  block_type=toreg
      settings: AttributesFormatString=<< %<shared_memory_name> >>  infoedit="Register block that writes data to a shared memory register.  Delay of one sample period."  block_version=12.3
  To Register7 : xbsIndex_r4/To Register  shared_memory_name='register04rv'  init=0  ownership=Locally owned and initialized  explicit_data_type=off  gui_display_data_type=Fixed-point  arith_type="Signed  (2's comp)"  n_bits=16  bin_pt=14  preci_type=Single  dbl_ovrd=off  block_type=toreg
      settings: AttributesFormatString=<< %<shared_memory_name> >>  infoedit="Register block that writes data to a shared memory register.  Delay of one sample period."  block_version=12.3
  To Register8 : xbsIndex_r4/To Register  shared_memory_name='register05rd'  init=0  ownership=Locally owned and initialized  explicit_data_type=off  gui_display_data_type=Fixed-point  arith_type="Signed  (2's comp)"  n_bits=16  bin_pt=14  preci_type=Single  dbl_ovrd=off  block_type=toreg
      settings: AttributesFormatString=<< %<shared_memory_name> >>  infoedit="Register block that writes data to a shared memory register.  Delay of one sample period."  block_version=12.3
  To Register9 : xbsIndex_r4/To Register  shared_memory_name='register06rd'  init=0  ownership=Locally owned and initialized  explicit_data_type=off  gui_display_data_type=Fixed-point  arith_type="Signed  (2's comp)"  n_bits=16  bin_pt=14  preci_type=Single  dbl_ovrd=off  block_type=toreg
      settings: AttributesFormatString=<< %<shared_memory_name> >>  infoedit="Register block that writes data to a shared memory register.  Delay of one sample period."  block_version=12.3
  rst_i : xbsIndex_r4/Gateway In  gui_display_data_type=Fixed-point  arith_type=Boolean  n_bits=1  bin_pt=0  preci_type=Single  exp_width=8  frac_width=24  quantization="Round  (unbiased: +/- Inf)"  overflow=Saturate  period=USER_TS  dbl_ovrd=off  timing_constraint=None  locs_specified=off  LOCs={}  hdl_port=on  block_type=gatewayin
      settings: infoedit="Gateway in block.  Converts inputs of type Simulink integer, double and fixed point to  Xilinx fixed point or floating-point data type.<br><br>Hardware notes:  In hardware these blocks become top level input ports."  block_version=12.3
  rst_o : xbsIndex_r4/Gateway Out  hdl_port=on  timing_constraint=None  locs_specified=off  LOCs={}  block_type=gatewayout
      settings: infoedit="Gateway out block.  Converts Xilinx fixed point or floating-point type inputs into ouputs of type Simulink integer, double, or fixed point.<br><br>Hardware notes:  In hardware these blocks become top level output ports or are discarded, depending on how they are configured."  block_version=12.3
  tx_en_in{1,3..9,11..31,38..43,51..52,58..62,65,67,75,86..87,89..90,92..100,104..105,107,109,113..114,116..117,119..121,123..125,127..128} (74 alike) : xbsIndex_r4/Register  init=0  rst=off  en=off  dbl_ovrd=off  block_type=register
  tx_en_in{2,10,33,50,53..54,66,122,126} (9 alike) : xbsIndex_r4/Register  init=0  rst=on  en=on  dbl_ovrd=off  block_type=register
  tx_en_in108 : xbsIndex_r4/Register  init=0  rst=off  en=on  dbl_ovrd=off  block_type=register
  tx_en_in115 : xbsIndex_r4/Register  init=200000 - 29  rst=on  en=on  dbl_ovrd=off  block_type=register
  tx_en_in118 : xbsIndex_r4/Register  init=19136  rst=on  en=on  dbl_ovrd=off  block_type=register
  tx_en_in85 : xbsIndex_r4/Register  init=1  rst=on  en=on  dbl_ovrd=off  block_type=register
  tx_en_in88 : xbsIndex_r4/Register  init=hex2dec('80000000')  rst=on  en=on  dbl_ovrd=off  block_type=register
  tx_en_in91 : xbsIndex_r4/Register  init=hex2dec('00000000')  rst=on  en=on  dbl_ovrd=off  block_type=register
  user_int_1o : xbsIndex_r4/Gateway Out  hdl_port=on  timing_constraint=None  locs_specified=off  LOCs={}  block_type=gatewayout
      settings: infoedit="Gateway out block.  Converts Xilinx fixed point or floating-point type inputs into ouputs of type Simulink integer, double, or fixed point.<br><br>Hardware notes:  In hardware these blocks become top level output ports or are discarded, depending on how they are configured."  block_version=12.3
  user_int_2o : xbsIndex_r4/Gateway Out  hdl_port=on  timing_constraint=None  locs_specified=off  LOCs={}  block_type=gatewayout
      settings: infoedit="Gateway out block.  Converts Xilinx fixed point or floating-point type inputs into ouputs of type Simulink integer, double, or fixed point.<br><br>Hardware notes:  In hardware these blocks become top level output ports or are discarded, depending on how they are configured."  block_version=12.3
  user_int_3o : xbsIndex_r4/Gateway Out  hdl_port=on  timing_constraint=None  locs_specified=off  LOCs={}  block_type=gatewayout
      settings: infoedit="Gateway out block.  Converts Xilinx fixed point or floating-point type inputs into ouputs of type Simulink integer, double, or fixed point.<br><br>Hardware notes:  In hardware these blocks become top level output ports or are discarded, depending on how they are configured."  block_version=12.3
  wires:
  rst_i/1 -> Inverter3/1
  tx_en_in26/1 -> rst_o/1  "rst"
  Constant2/1 -> tx_en_in18/1
  BRAM_rd_dout/1 -> tx_en_in20/1, tx_en_in14/1  "BRAM_data"
  Counter4/1 -> tx_en_in17/1, tx_en_in15/1
  tx_en_in17/1 -> tx_en_in30/1
  tx_en_in30/1 -> tx_en_in16/1
  tx_en_in38/1 -> FIFO_wr_din/1
  From Register3/1 -> tx_en_in9/1
  From Register4/1 -> tx_en_in4/1
  From Register7/1 -> tx_en_in12/1
  From Register8/1 -> tx_en_in8/1
  tx_en_in4/1 -> Convert3/1
  tx_en_in8/1 -> Convert9/1
  tx_en_in2/1 -> To Register/1  "reg01"
  tx_en_in1/1 -> To Register1/1
  tx_en_in10/1 -> To Register3/1  "reg03"
  tx_en_in7/1 -> To Register5/1
  From Register9/1 -> tx_en_in62/1
  From Register10/1 -> tx_en_in58/1
  From Register11/1 -> tx_en_in60/1
  From Register12/1 -> tx_en_in59/1
  From Register13/1 -> tx_en_in52/1
  From Register14/1 -> tx_en_in61/1
  tx_en_in62/1 -> tx_en_in50/1  "dinb"
  tx_en_in58/1 -> Convert5/1
  tx_en_in60/1 -> tx_en_in53/1
  tx_en_in59/1 -> Convert6/1
  tx_en_in52/1 -> tx_en_in54/1
  tx_en_in61/1 -> Convert7/1
  tx_en_in50/1 -> To Register6/1  "Thread1_reg"
  tx_en_in53/1 -> To Register8/1  "Thread2_reg"
  tx_en_in54/1 -> To Register9/1  "NewBurst_reg"
  Constant6/1 -> To Register6/2, To Register8/2, To Register9/2, To Register11/2, To Register15/2, To Register14/2, To Register17/2, To Register16/2, To Register19/2, To Register18/2, To Register21/2, To Register20/2, To Register23/2, To Register22/2, To Register25/2, To Register24/2, To Register27/2, To Register26/2, To Register13/2, To Register12/2, To Register/2, To Register1/2, To Register3/2, To Register5/2, To Register10/2, To Register7/2, To Register4/2, To Register2/2
  Convert5/1 -> tx_en_in50/3, tx_en_in95/1
  Convert6/1 -> tx_en_in53/3, tx_en_in96/1
  Convert7/1 -> tx_en_in54/3, tx_en_in97/1
  From Register15/1 -> ?
  From Register16/1 -> ?
  Constant20/1 -> tx_en_in54/2
  Constant25/1 -> tx_en_in50/2
  Constant24/1 -> tx_en_in53/2
  From Register17/1 -> tx_en_in65/1
  From Register18/1 -> tx_en_in67/1
  tx_en_in65/1 -> tx_en_in66/1
  tx_en_in67/1 -> Convert8/1
  Convert8/1 -> tx_en_in66/3, tx_en_in13/1
  tx_en_in3/1 -> user_int_1o/1
  tx_en_in75/1 -> user_int_2o/1
  From Register5/1 -> tx_en_in6/1
  From Register6/1 -> tx_en_in5/1
  tx_en_in6/1 -> tx_en_in33/1
  tx_en_in5/1 -> Convert1/1
  Convert1/1 -> tx_en_in33/3, tx_en_in94/1
  Constant26/1 -> tx_en_in33/2
  tx_en_in33/1 -> To Register2/1  "ChunkDMAinProgress"
  tx_en_in66/1 -> To Register13/1  "ResetIRQ_reg"
  tx_en_in51/1 -> user_int_3o/1
  From Register20/1 -> tx_en_in87/1
  From Register21/1 -> tx_en_in86/1
  tx_en_in87/1 -> tx_en_in85/1
  tx_en_in86/1 -> Convert4/1
  tx_en_in85/1 -> To Register15/1  "Thread2_reg"
  Convert4/1 -> tx_en_in85/3, tx_en_in98/1
  Constant7/1 -> tx_en_in85/2
  From Register22/1 -> tx_en_in90/1
  From Register23/1 -> tx_en_in89/1
  tx_en_in90/1 -> tx_en_in88/1
  tx_en_in89/1 -> Convert11/1
  tx_en_in88/1 -> To Register17/1  "Thread2_reg"
  Convert11/1 -> tx_en_in88/3, tx_en_in99/1
  Constant4/1 -> tx_en_in88/2
  From Register24/1 -> tx_en_in93/1
  From Register25/1 -> tx_en_in92/1
  tx_en_in93/1 -> tx_en_in91/1
  tx_en_in92/1 -> Convert12/1
  tx_en_in91/1 -> To Register19/1  "Thread2_reg"
  Convert12/1 -> tx_en_in91/3, tx_en_in100/1
  Constant9/1 -> tx_en_in91/2
  tx_en_in94/1 -> To Register4/1
  tx_en_in95/1 -> To Register7/1
  tx_en_in96/1 -> To Register10/1
  tx_en_in97/1 -> To Register11/1
  tx_en_in98/1 -> To Register14/1
  tx_en_in99/1 -> To Register16/1
  tx_en_in100/1 -> To Register18/1
  Constant12/1 -> tx_en_in66/2
  FIFO_rd_pempty/1 -> tx_en_in39/1, tx_en_in25/1  "FIFO_rd_pempty"
  FIFO_rd_count/1 -> tx_en_in40/1, tx_en_in27/1  "FIFO_rd_count"
  FIFO_wr_full/1 -> tx_en_in41/1, tx_en_in28/1  "FIFO_wr_full"
  FIFO_wr_pfull/1 -> tx_en_in42/1, tx_en_in29/1  "FIFO_wr_pfull"
  FIFO_rd_dout/1 -> tx_en_in38/1, tx_en_in24/1  "FIFO_data_in/out"
  tx_en_in15/1 -> BRAM_rd_addr/1
  tx_en_in16/1 -> tx_en_in19/1, tx_en_in11/1  "BRAM_addr"
  tx_en_in18/1 -> tx_en_in43/1
  tx_en_in19/1 -> BRAM_wr_addr/1
  tx_en_in20/1 -> BRAM_wr_din/1
  tx_en_in43/1 -> BRAM_wr_en/1
  Inverter3/1 -> tx_en_in26/1
  FIFO_wr_count/1 -> tx_en_in104/1, tx_en_in31/1  "FIFO_wr_count"
  FIFO_rd_valid/1 -> tx_en_in109/1, tx_en_in23/1  "FIFO_wr_en"
  tx_en_in108/1 -> FIFO_rd_en/1
  Constant15/1 -> Logical4/1
  tx_en_in109/1 -> FIFO_wr_en/1
  Logical4/1 -> tx_en_in108/1, tx_en_in22/1  "FIFO_rd_en"
  FIFO_rd_empty/1 -> tx_en_in105/1
  Inverter5/1 -> Logical4/2
  From Register26/1 -> tx_en_in117/1
  From Register27/1 -> tx_en_in116/1
  tx_en_in117/1 -> tx_en_in115/1
  tx_en_in116/1 -> Convert14/1
  tx_en_in115/1 -> To Register21/1  "Thread2_reg"
  Convert14/1 -> tx_en_in115/3, tx_en_in113/1
  Constant19/1 -> tx_en_in115/2
  tx_en_in113/1 -> To Register20/1
  From Register28/1 -> tx_en_in120/1
  From Register29/1 -> tx_en_in119/1
  tx_en_in120/1 -> tx_en_in118/1
  tx_en_in119/1 -> Convert15/1
  tx_en_in118/1 -> To Register23/1  "Thread2_reg"
  Convert15/1 -> tx_en_in114/1, tx_en_in118/3
  Constant21/1 -> tx_en_in118/2
  tx_en_in114/1 -> To Register22/1
  From Register30/1 -> tx_en_in124/1
  From Register31/1 -> tx_en_in123/1
  tx_en_in124/1 -> tx_en_in122/1
  tx_en_in123/1 -> Convert16/1
  tx_en_in122/1 -> To Register25/1  "Thread2_reg"
  Convert16/1 -> tx_en_in122/3, tx_en_in121/1
  Constant22/1 -> tx_en_in122/2
  tx_en_in121/1 -> To Register24/1
  From Register32/1 -> tx_en_in128/1
  From Register33/1 -> tx_en_in127/1
  tx_en_in128/1 -> tx_en_in126/1
  tx_en_in127/1 -> Convert17/1
  tx_en_in126/1 -> To Register27/1  "Thread2_reg"
  Convert17/1 -> tx_en_in125/1, tx_en_in126/3
  Constant23/1 -> tx_en_in126/2
  tx_en_in125/1 -> To Register26/1
  Constant14/1 -> tx_en_in108/2
  tx_en_in13/1 -> To Register12/1
  Constant8/1 -> tx_en_in3/1
  Constant10/1 -> tx_en_in75/1
  Constant11/1 -> tx_en_in51/1
  Convert3/1 -> tx_en_in1/1, tx_en_in2/3  "TimeCountReset"
  Constant1/1 -> tx_en_in2/2
  Convert9/1 -> tx_en_in10/3, tx_en_in7/1  "TimeCountTrigger"
  Constant3/1 -> tx_en_in10/2
  tx_en_in12/1 -> tx_en_in10/1
  tx_en_in9/1 -> tx_en_in2/1  "dinb"
  tx_en_in105/1 -> tx_en_in107/1, tx_en_in21/1  "FIFO_empty"
  tx_en_in107/1 -> Inverter5/1
  tx_en_in11/1 -> ChipScope/1  "BRAM_addr"
  tx_en_in14/1 -> ChipScope/2  "BRAM_data"
  tx_en_in21/1 -> ChipScope/3  "FIFO_empty"
  tx_en_in22/1 -> ChipScope/4  "FIFo_rd_en"
  tx_en_in23/1 -> ChipScope/5  "FIFO_wr_en"
  tx_en_in24/1 -> ChipScope/6  "FIFO_data_in/out"
  tx_en_in25/1 -> ChipScope/7  "FIFO_rd_pempty"
  tx_en_in27/1 -> ChipScope/8  "FIFO_rd_count"
  tx_en_in28/1 -> ChipScope/9  "FIFO_wr_full"
  tx_en_in29/1 -> ChipScope/10  "FIFO_wr_pfull"
  tx_en_in31/1 -> ChipScope/11  "FIFO_wr_count"
